simulink model "Refined_Model_40"  (R2020b)
settings: Solver=FixedStepAuto  StartTime=0.0  StopTime=5000  FixedStep=0.1  RelTol=1e-3
values from neighbouring files (symbols this model uses):
  ALInpSpeed = AxlLoss (1,:)    [GPS_val.m]    (also in ICEBEV_Script.m; ICEBEV_Script_VECTO.m; ICE_Script.m; ICE_Script_SSVal.m)
  ALInpTor = AxlLoss(:,1)    [GPS_val.m]    (also in ICEBEV_Script.m; ICEBEV_Script_VECTO.m; ICE_Script.m; ICE_Script_SSVal.m)
  ALTableVal = AxlLoss(2:end,2:end)    [GPS_val.m]    (also in ICEBEV_Script.m; ICEBEV_Script_VECTO.m; ICE_Script.m; ICE_Script_SSVal.m)
  CovDist = RoadProfile(:,4)    [ICE_Val.m]
  Cx = VehicleDefine(7,3)    [BEV_Basictest.m]    (also in GPS_val.m; ICEBEV_Script.m; ICEBEV_Script_VECTO.m; ICE_Script.m)
  Dist = 1:length(MaxSpeedProfile)    [GPS_val.m]    (also in ICE_Script.m; ICE_Val.m = [1:CovDist(end)])
  DynRolRad = VehicleDefine(5,3)    [BEV_Basictest.m]    (also in GPS_val.m; ICEBEV_Script.m; ICEBEV_Script_VECTO.m; ICE_Script.m)
  FDR = VehicleDefine(20,3)    [BEV_Basictest.m]    (also in GPS_val.m = VehicleDefine(22,3); ICEBEV_Script.m = VehicleDefine(22,3); ICEBEV_Script_VECTO.m = VehicleDefine(22,3); ICE_Script.m = VehicleDefine(22,3))
  Fr = VehicleDefine(13,3)    [BEV_Basictest.m]    (also in GPS_val.m; ICEBEV_Script.m; ICEBEV_Script_VECTO.m; ICE_Script.m)
  g = VehicleDefine(14,3)    [BEV_Basictest.m]    (also in GPS_val.m; ICEBEV_Script.m; ICEBEV_Script_VECTO.m; ICE_Script.m)
  GNo = GBXDefine(:,1)    [GPS_val.m]    (also in ICEBEV_Script.m; ICEBEV_Script_VECTO.m; ICE_Script.m; ICE_Script_SSVal.m)
  IntpSlope = round(IntpSlope,1)    [GPS_val.m]    (also in ICE_Script.m; ICE_Val.m = A)
  Jk = VehicleDefine(15,3)    [BEV_Basictest.m]    (also in GPS_val.m; ICEBEV_Script.m; ICEBEV_Script_VECTO.m; ICE_Script.m)
  MaxAcc = 1    [BEV_Basictest.m]    (also in GPS_val.m; ICEBEV_Script.m; ICEBEV_Script_VECTO.m; ICE_Script.m)
  MaxDec = 1    [BEV_Basictest.m]    (also in GPS_val.m; ICEBEV_Script.m; ICEBEV_Script_VECTO.m; ICE_Script.m)
  MaxSpeedProfile = FMSP    [GPS_val.m]    (also in ICE_Script.m; ICE_Val.m = repelem(SegSPLatinmps,SegLeninm))
  Me = VehicleDefine(10,3)    [BEV_Basictest.m]    (also in GPS_val.m; ICEBEV_Script.m; ICEBEV_Script_VECTO.m; ICE_Script.m)
  Mt = VehicleDefine(12,3)    [BEV_Basictest.m]    (also in GPS_val.m; ICEBEV_Script.m; ICEBEV_Script_VECTO.m; ICE_Script.m)
  Mtot = Mv+Me+Mt    [BEV_Basictest.m]    (also in GPS_val.m; ICEBEV_Script.m; ICEBEV_Script_VECTO.m; ICE_Script.m)
  Mv = VehicleDefine(9,3)    [BEV_Basictest.m]    (also in GPS_val.m; ICEBEV_Script.m; ICEBEV_Script_VECTO.m; ICE_Script.m)
  NoSteps = round(Dist(end))    [GPS_val.m]    (also in ICE_Script.m; ICE_Val.m = 3002)
  NoWhlFA = VehicleDefine(2,3)    [BEV_Basictest.m]    (also in GPS_val.m; ICE_Script.m; ICE_Val.m; ICE_Val_new.m)
  NoWhlRA = VehicleDefine(4,3)    [BEV_Basictest.m]    (also in GPS_val.m; ICE_Script.m; ICE_Val.m; ICE_Val_new.m)
  rho = VehicleDefine(6,3)    [BEV_Basictest.m]    (also in GPS_val.m; ICEBEV_Script.m; ICEBEV_Script_VECTO.m; ICE_Script.m)
  s = divisors(length(MaxSpeedProfile))    [GPS_val.m]    (also in ICEBEV_Script.m = round(FLoadTor); ICEBEV_Script_VECTO.m = round(FLoadTor); ICE_Script.m = round(FLoadTor); ICE_Script_SSVal.m = round(FLoadTor))
  SegNo = RoadProfile(:,1)    [ICE_Val.m]
  SegSPLatinmps = (sqrt(aMaxLat*g*CurRadinm))    [GPS_val.m]    (also in ICE_Script.m; ICE_Val.m)
  Sx = VehicleDefine(8,3)    [BEV_Basictest.m]    (also in GPS_val.m; ICEBEV_Script.m; ICEBEV_Script_VECTO.m; ICE_Script.m)
undefined symbols (not defined in the file or in its folder): G1Inprpm, Gmot, Jgbx, Stoptimes
libraries: autolibshared x2, vehdynlibtire x2, autolibdatasheetbattery x1, autolibmappedmotor x1
(part 3 of 3)

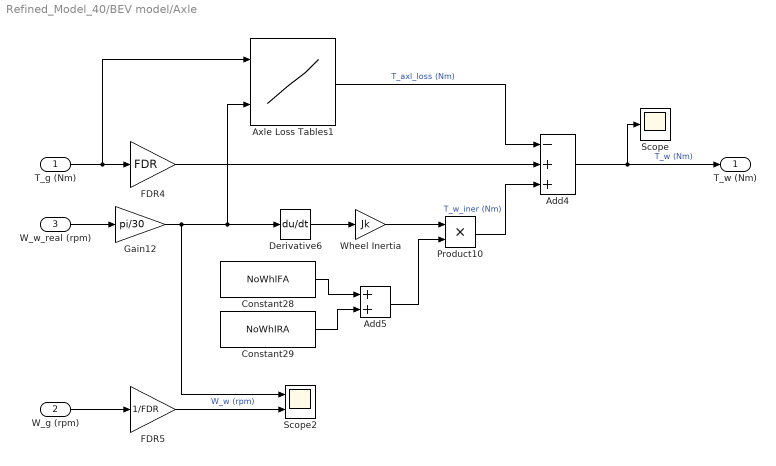
== system Refined_Model_40/BEV model/Axle ==
  T_g (Nm) : Inport
  W_g (rpm) : Inport  Port=2
  W_w_real (rpm) : Inport  Port=3
  Add4 : Sum  Inputs=-++
  Add5 : Sum
  Axle Loss Tables1 : Lookup_n-D  BreakpointsForDimension1=ALInpTor  BreakpointsForDimension2=ALInpSpeed  BreakpointsForDimension3=GNo  Table=ALTableVal  InterpMethod=Linear Lagrange  InternalRulePriority=Speed  RndMeth=Simplest  InputSameDT=on
      settings: InputPortMap=u0,u1
  Constant28 : Constant  Value=NoWhlFA
  Constant29 : Constant  Value=NoWhlRA
  Derivative6 : Derivative
  FDR4 : Gain  Gain=FDR
  FDR5 : Gain  Gain=1/FDR
  Gain12 : Gain  Gain=pi/30
  Product10 : Product
  Scope : Scope
  Scope2 : Scope  NumInputPorts=2
  Wheel Inertia : Gain  Gain=Jk
  T_w (Nm) : Outport
  wires:
  Product10/1 -> Add4/3  "T_w_iner (Nm)"
  Derivative6/1 -> Wheel Inertia/1
  Add5/1 -> Product10/2
  Constant29/1 -> Add5/2
  Constant28/1 -> Add5/1
  FDR4/1 -> Add4/2
  FDR5/1 -> Scope2/2  "W_w (rpm)"
  Wheel Inertia/1 -> Product10/1
  Add4/1 -> T_w (Nm)/1, Scope/1  "T_w (Nm)"
  T_g (Nm)/1 -> Axle Loss Tables1/1, FDR4/1
  W_g (rpm)/1 -> FDR5/1
  W_w_real (rpm)/1 -> Gain12/1
  Axle Loss Tables1/1 -> Add4/1  "T_axl_loss (Nm)"
  Gain12/1 -> Scope2/1, Axle Loss Tables1/2, Derivative6/1

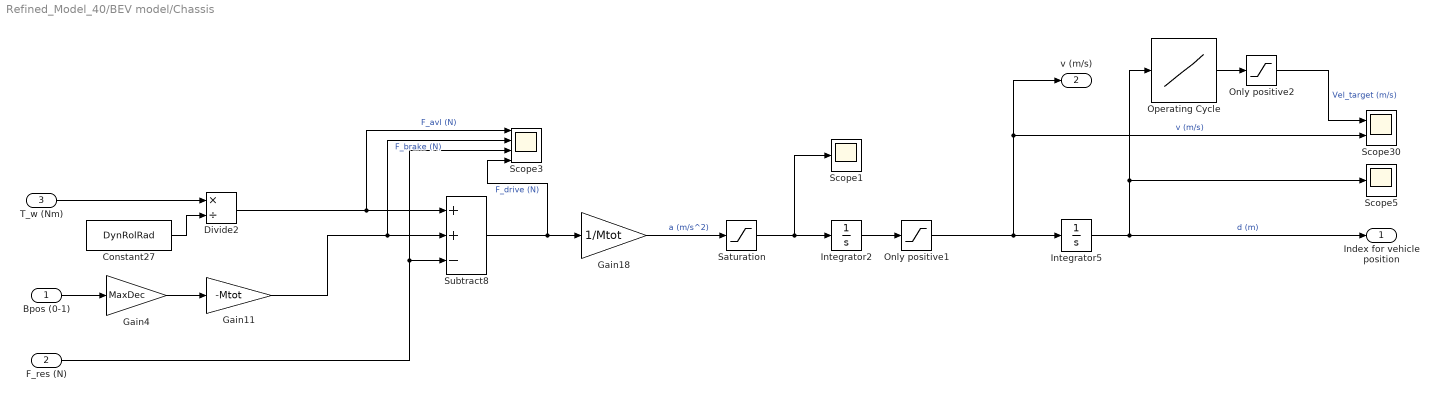
== system Refined_Model_40/BEV model/Chassis ==
  Bpos (0-1) : Inport
  F_res (N) : Inport  Port=2
  T_w (Nm) : Inport  Port=3
  Constant27 : Constant  Value=DynRolRad
  Divide2 : Product  Inputs=*/
  Gain11 : Gain  Gain=-Mtot
  Gain18 : Gain  Gain=1/Mtot
  Gain4 : Gain  Gain=MaxDec
  Integrator2 : Integrator  ContinuousStateAttributes='acceleration'
  Integrator5 : Integrator  ContinuousStateAttributes='velocity'
  Only positive1 : Saturate  UpperLimit=inf  LowerLimit=0
  Only positive2 : Saturate  UpperLimit=inf  LowerLimit=0
  Operating Cycle : Lookup_n-D  NumberOfTableDimensions=1  BreakpointsForDimension1=Dist  BreakpointsForDimension2=G1Inprpm  Table=MaxSpeedProfile  InterpMethod=Linear Lagrange  InternalRulePriority=Speed  RndMeth=Simplest  InputSameDT=on
  Saturation : Saturate  UpperLimit=MaxAcc  LowerLimit=-(MaxDec)
  Scope1 : Scope
  Scope3 : Scope  NumInputPorts=4
  Scope30 : Scope  NumInputPorts=2
  Scope5 : Scope
  Subtract8 : Sum  Inputs=++-
  Index for vehicle position : Outport
  v (m/s) : Outport  Port=2
  wires:
  Constant27/1 -> Divide2/2
  Subtract8/1 -> Scope3/4, Gain18/1  "F_drive (N)"
  Divide2/1 -> Subtract8/1, Scope3/1  "F_avl (N)"
  Integrator5/1 -> Index for vehicle position/1, Scope5/1, Operating Cycle/1  "d (m)"
  Integrator2/1 -> Only positive1/1
  T_w (Nm)/1 -> Divide2/1
  Gain11/1 -> Subtract8/2, Scope3/2  "F_brake (N)"
  Only positive1/1 -> v (m/s)/1, Scope30/2, Integrator5/1  "v (m/s)"
  Operating Cycle/1 -> Only positive2/1
  Gain18/1 -> Saturation/1  "a (m/s^2)"
  Bpos (0-1)/1 -> Gain4/1
  Gain4/1 -> Gain11/1
  F_res (N)/1 -> Subtract8/3, Scope3/3
  Saturation/1 -> Integrator2/1, Scope1/1
  Only positive2/1 -> Scope30/1  "Vel_target (m/s)"

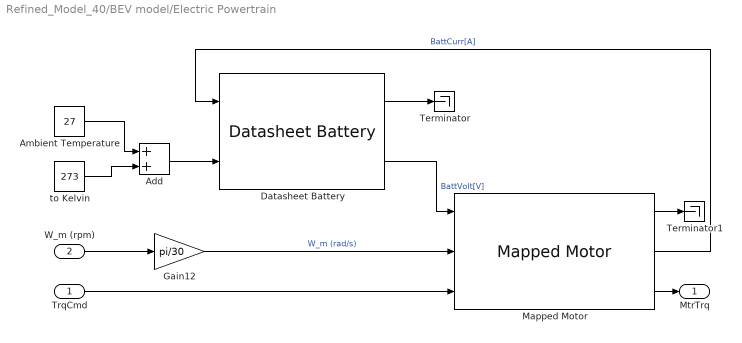
== system Refined_Model_40/BEV model/Electric Powertrain ==
  TrqCmd : Inport
  W_m (rpm) : Inport  Port=2
  Add : Sum
  Ambient Temperature : Constant  Value=27
  Datasheet Battery : autolibdatasheetbattery/Datasheet Battery  CapacityCtrl=Parameter  OutputVlt=Unfiltered  BattChargeMax=400  Em=[2.8 3.228 3.284 3.361 3.408 3.427 3.472 3.477 3.493 3.504 3.516 3.528 3.537 3.545 3.555 3.561 3.566 3.576 3.587 3.589 3.594 3.6 3.608 3.61 3.616 3.619 3.626 3.632 3.637 3.64 3.645 3.646 3.652 3.655 3.658 3.661 3.664 3.668 3.673 3.678 3.68 3.681 3.686 3.692 3.699 3.702 3.705 3.71 3.717 3.723 3.728 3.733 3.735 3.742 3.749 3.755 3.761 3.768 3.773 3.78 3.791 3.798 3.798 3.814 3.818 3.825 3.841 3.846 3.855 3.863 3.877 3.885 3.894 3.907 3.919 3.926 3.935 3.944 3.954 3.964 3.974 3.988 3.998 4.014 4.029 4.034 4.047 4.065 4.074 4.086 4.097 4.131 4.126 4.138 4.15 4.18 4.174 4.187 4.207 4.231 4.221]  CapLUTBp=[0 0.01 0.02 0.03 0.04 0.05 0.06 0.07 0.08 0.09 0.1 0.11 0.12 0.13 0.14 0.15 0.16 0.17 0.18 0.19 0.2 0.21 0.22 0.23 0.24 0.25 0.26 0.27 0.28 0.29 0.3 0.31 0.32 0.33 0.34 0.35 0.36 0.37 0.38 0.39 0.4 0.41 0.42 0.43 0.44 0.45 0.46 0.47 0.48 0.49 0.5 0.51 0.52 0.53 0.54 0.55 0.56 0.57 0.58 0.59 0.6 0.61 0.62 0.63 0.64 0.65 0.66 0.67 0.68 0.69 0.7 0.71 0.72 0.73 0.74 0.75 0.76 0.77 0.78 0.79 0.8 0.81 0.82 0.83 0.84 0.85 0.86 0.87 0.88 0.89 0.9 0.91 0.92 0.93 0.94 0.95 0.96 0.97 0.98 0.99 1]  RInt=[0.008846 0.009319 0.009027 0.00847 0.01032 0.01314;0.006389 0.006554 0.005553 0.005525 0.006043 0.007805;0.004364 0.004101 0.00406 0.003452 0.003846 0.004517;0.002031 0.002563 0.002532 0.00246 0.002716 0.003047;0.001443 0.001825 0.001795 0.001778 0.001924 0.002234;0.0005603 0.0007192 0.0006887 0.0007557 0.0007355 0.001014;0.001028 0.001338 0.001 0.001536 0.001546 0.002789]  BattTempBp=[243.1 253.1 263.1 273.1 283.1 298.1 313.1]  CapSOCBp=[0 0.2 0.4 0.6 0.8 1]  Ns=1  Np=1  BattCapInit=400  Tc=1/1000  Vinit=4.221  RefBlkName='autolibdatasheetbattery/Datasheet Battery'
      settings: SourceProductBaseCode=PW
  Gain12 : Gain  Gain=pi/30
  Mapped Motor : autolibmappedmotor/Mapped Motor  port_config=Speed  param_by=Maximum torque and power  w_t=[ 0 375 750 800 ]  T_t=[0.09 0.08 0.07 0]  torque_max=2200  power_max=295000  Tc=0.02  param_loss=Single efficiency measurement  eff=100  w_eff=375  T_eff=0.08  Piron=0  Pbase=0  w_eff_bp=[-8000 -4000 0 4000 8000]  T_eff_bp=[0 0.03 0.06 0.09]  Temp_eff_bp=[233.15 293.15 373.15]  losses_table=[1.49 1.67 2.21 3.10; 0.42 0.69 1.14 2.03; 0.06 0.24 0.78 1.68; 0.42 0.69 1.14 2.03; 1.49 1.67 2.21 3.10]  losses_table_3d=cat(3,1.05*[1.49 1.67 2.21 3.10; 0.42 0.69 1.14 2.03; 0.06 0.24 0.78 1.68; 0.42 0.69 1.14 2.03; 1.49 1.67 2.21 3.10],[1.49 1.67 2.21 3.10; 0.42 0.69 1.14 2.03; 0.06 0.24 0.78 1.68; 0.42 0.69 1.14 2.03; 1.49 1.67 2.21 3.10],1.03*[1.49 1.67 2.21 3.10; 0.42 0.69 1.14 2.03; 0.06 0.24 0.78 1.68; 0.42 0.69 1.14 2.03; 1.49 1.67 2.21 3.10])  efficiency_table=[95 95 95 95; 95 95 95 95; 95 95 95 95; 95 95 95 95; 95 95 95 95]  efficiency_table_3d=cat(3,90*ones(5,4),95*ones(5,4),92*ones(5,4))  J=5e-6  b=1e-5  omega_o=0  T_t_extended=[0 0.07 0.08 0.09 0.08 0.07 0]  w_t_extended=[-800 -750 -375 0 375 750 800]  KLossIron=0  KLossCopper=0  x_w_eff_vec=[-8000 -4000 0 4000 8000]  x_T_eff_vec=[-0.09 -0.06 -0.03 0 0.03 0.06 0.09]  x_tmp_eff_vec=[233.15 293.15 373.15]  x_losses_mat=[3.1 2.21 1.67 1.49 1.67 2.21 3.1;2.03 1.14 0.69 0.42 0.69 1.14 2.03;1.68 0.78 0.24 0.06 0.24 0.78 1.68;2.03 1.14 0.69 0.42 0.69 1.14 2.03;3.1 2.21 1.67 1.49 1.67 2.21 3.1]  x_losses_mat_3d=cat(3,[3.255 2.3205 1.7535 1.5645 1.7535 2.3205 3.255;2.1315 1.197 0.7245 0.441 0.7245 1.197 2.1315;1.764 0.819 0.252 0.063 0.252 0.819 1.764;2.1315 1.197 0.7245 0.441 0.7245 1.197 2.1315;3.255 2.3205 1.7535 1.5645 1.7535 2.3205 3.255],[3.1 2.21 1.67 1.49 1.67 2.21 3.1;2.03 1.14 0.69 0.42 0.69 1.14 2.03;1.68 0.78 0.24 0.06 0.24 0.78 1.68;2.03 1.14 0.69 0.42 0.69 1.14 2.03;3.1 2.21 1.67 1.49 1.67 2.21 3.1],[3.193 2.2763 1.7201 1.5347 1.7201 2.2763 3.193;2.0909 1.1742 0.7107 0.4326 0.7107 1.1742 2.0909;1.7304 0.8034 0.2472 0.0618 0.2472 0.8034 1.7304;2.0909 1.1742 0.7107 0.4326 0.7107 1.1742 2.0909;3.193 2.2763 1.7201 1.5347 1.7201 2.2763 3.193])  CalLossMapData={}  CalLossWithTempMapData={}  aMode=2  RefBlkName='autolibmappedmotor/Mapped Motor'
      settings: SourceProductBaseCode=PW,MT,UV,VE,VP
  Terminator : Terminator
  Terminator1 : Terminator
  to Kelvin : Constant  Value=273
  MtrTrq : Outport
  wires:
  Mapped Motor/3 -> MtrTrq/1
  Ambient Temperature/1 -> Add/1
  Datasheet Battery/2 -> Mapped Motor/1  "BattVolt[V]"
  W_m (rpm)/1 -> Gain12/1
  Mapped Motor/2 -> Datasheet Battery/1  "BattCurr[A]"
  to Kelvin/1 -> Add/2
  Add/1 -> Datasheet Battery/2
  TrqCmd/1 -> Mapped Motor/3
  Gain12/1 -> Mapped Motor/2  "W_m (rad/s)"
  Datasheet Battery/1 -> Terminator/1
  Mapped Motor/1 -> Terminator1/1

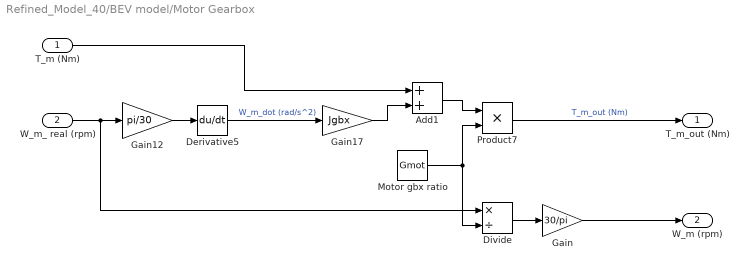
== system Refined_Model_40/BEV model/Motor Gearbox ==
  T_m (Nm) : Inport
  W_m_ real (rpm) : Inport  Port=2
  Add1 : Sum
  Derivative5 : Derivative
  Divide : Product  Inputs=*/
  Gain : Gain  Gain=30/pi
  Gain12 : Gain  Gain=pi/30
  Gain17 : Gain  Gain=Jgbx
  Motor gbx ratio : Constant  Value=Gmot
  Product7 : Product
  T_m_out (Nm) : Outport
  W_m (rpm) : Outport  Port=2
  wires:
  Motor gbx ratio/1 -> Product7/2, Divide/2
  Divide/1 -> Gain/1
  Gain/1 -> W_m (rpm)/1
  W_m_ real (rpm)/1 -> Divide/1, Gain12/1
  Add1/1 -> Product7/1
  Derivative5/1 -> Gain17/1  "W_m_dot (rad/s^2)"
  Gain17/1 -> Add1/2
  Product7/1 -> T_m_out (Nm)/1  "T_m_out (Nm)"
  T_m (Nm)/1 -> Add1/1
  Gain12/1 -> Derivative5/1

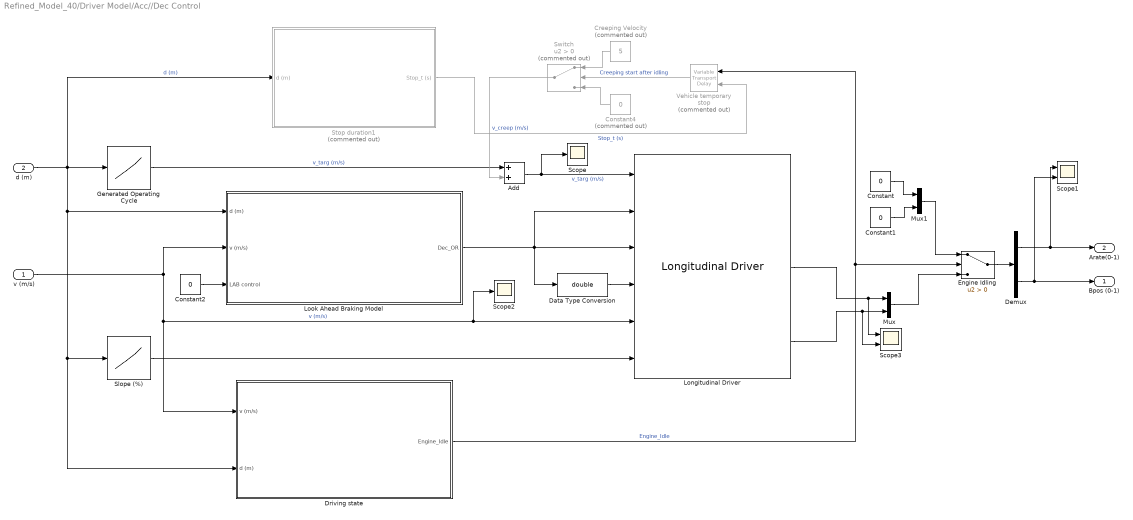
== system Refined_Model_40/Driver Model/Acc//Dec Control ==
  v (m/s) : Inport
  d (m) : Inport  Port=2
  Add : Sum
  Constant : Constant  Value=0
  Constant1 : Constant  Value=0
  Constant2 : Constant  Value=0
  Constant4 : Constant  Commented=on  Value=0
  Creeping Velocity : Constant  Commented=on  Value=5
  Data Type Conversion : DataTypeConversion  OutDataTypeStr=double
  Demux : Demux  Outputs=2
  Driving state : Subsystem
  Engine Idling : Switch  Criteria=u2 > Threshold
  Generated Operating Cycle : Lookup_n-D  NumberOfTableDimensions=1  BreakpointsForDimension1=Dist  BreakpointsForDimension2=G1Inprpm  Table=MaxSpeedProfile  InterpMethod=Linear Lagrange  InternalRulePriority=Speed  RndMeth=Simplest  InputSameDT=on
  Longitudinal Driver : autolibshared/Longitudinal Driver  extAccelOvr=off  extDecelOvr=on  extAccelHld=off  extDecelHld=off  extAccelZero=on  extDecelZero=off  cntrlType=PI  shftType=None  velUnits=m/s  gearOut=off  Kp=1  Ki=1  Kff=0  Kg=0  VehVelVec=[0 100]  KffVec=[.1 .1]  KpVec=[10 10]  KiVec=[5 5]  KgVec=[0 0]  m=1500  Kpt=3000  tau=.1  L=2  aR=200  bR=2.5  cR=.5  g=9.81  vnom=100  Kaw=0  tauerr=0  tauPt=2  GearInit=0  tShift=.1  pdlVec=[0.1 0.4 0.5 0.9]  upShftTbl=[-1 12.9375 26.4375 39.9375 51.18749999999999 62.4375 72.84375 83.25;-1 16.3125 29.8125 43.3125 54.5624 65.8125 76.78125 87.75;-1 19.6875 33.1875 46.68749999999999 57.9375 69.1875 80.71875 92.25;-1 33 52.5 77.25 100.5 138.75 161.875 185]  dwnShftTbl=[1 9.5625 23.0625 36.5625 47.8125 59.0625 68.90625 78.75;1 12.9375 26.4375 39.9375 51.18749999999999 62.4375 72.84375 83.25;1 16.3125 29.8125 43.3125 54.562499 65.8125 76.78125 87.75;1 19.6875 33.1875 46.68749999999999 57.9375 69.1875 80.71875 92.25]  tClutch=.5  tRev=.5  tPark=120  aMode=1  UpGearVec="[0  1  2  3  4  5  6  7]"  DownGearVec="[1  2  3  4  5  6  7  8]"
      settings: SourceProductBaseCode=PW,MT,UV,VE,VP
  Look Ahead Braking Model : Subsystem
  Mux : Mux  Inputs=2
  Mux1 : Mux  Inputs=2
  Scope : Scope
  Scope1 : Scope  NumInputPorts=2
  Scope2 : Scope
  Scope3 : Scope  NumInputPorts=2
  Slope (%) : Lookup_n-D  NumberOfTableDimensions=1  BreakpointsForDimension1=Dist  Table=IntpSlope  InternalRulePriority=Speed  RndMeth=Simplest  InputSameDT=on
  Stop duration1 : Subsystem  Commented=on
  Switch : Switch  Commented=on  Criteria=u2 > Threshold
  Vehicle temporary stop : VariableTransportDelay  Commented=on  VariableDelayType=Variable transport delay  MaximumDelay=10
  Bpos (0-1) : Outport
  Arate(0-1) : Outport  Port=2
  wires:
  Add/1 -> Scope/1, Longitudinal Driver/1  "v_targ (m/s)"
  Slope (%)/1 -> Longitudinal Driver/6
  Demux/1 -> Scope1/1, Arate(0-1)/1
  Demux/2 -> Bpos (0-1)/1, Scope1/2
  Constant/1 -> Mux1/1
  Mux/1 -> Engine Idling/3
  Constant1/1 -> Mux1/2
  Mux1/1 -> Engine Idling/1
  Engine Idling/1 -> Demux/1
  d (m)/1 -> Stop duration1/1(d (m)), Driving state/2(d (m)), Slope (%)/1, Look Ahead Braking Model/1(d (m)), Generated Operating Cycle/1  "d (m)"
  v (m/s)/1 -> Scope2/1, Longitudinal Driver/5, Driving state/1(v (m/s)), Look Ahead Braking Model/2(v (m/s))  "v (m/s)"
  Generated Operating Cycle/1 -> Add/1  "v_targ (m/s)"
  Data Type Conversion/1 -> Longitudinal Driver/4
  Longitudinal Driver/3 -> Scope3/2, Mux/2
  Stop duration1/1(Stop_t (s)) -> Vehicle temporary stop/2  "Stop_t (s)"
  Driving state/1(Engine_Idle) -> Vehicle temporary stop/1, Engine Idling/2  "Engine_Idle"
  Creeping Velocity/1 -> Switch/1
  Constant4/1 -> Switch/3
  Vehicle temporary stop/1 -> Switch/2  "Creeping start after idling"
  Switch/1 -> Add/2  "v_creep (m/s)"
  Look Ahead Braking Model/1(Dec_OR) -> Longitudinal Driver/2, Longitudinal Driver/3, Data Type Conversion/1
  Longitudinal Driver/2 -> Mux/1, Scope3/1
  Constant2/1 -> Look Ahead Braking Model/3(LAB control)

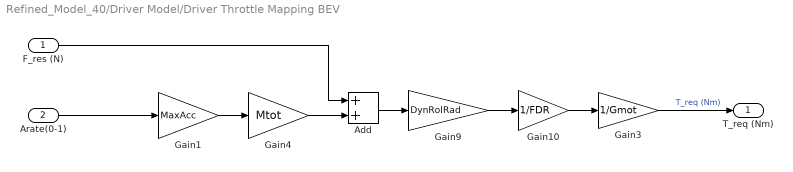
== system Refined_Model_40/Driver Model/Driver Throttle Mapping BEV ==
  F_res (N) : Inport
  Arate(0-1) : Inport  Port=2
  Add : Sum
  Gain1 : Gain  Gain=MaxAcc
  Gain10 : Gain  Gain=1/FDR
  Gain3 : Gain  Gain=1/Gmot
  Gain4 : Gain  Gain=Mtot
  Gain9 : Gain  Gain=DynRolRad
  T_req (Nm) : Outport
  wires:
  Gain3/1 -> T_req (Nm)/1  "T_req (Nm)"
  Gain1/1 -> Gain4/1
  Gain9/1 -> Gain10/1
  Add/1 -> Gain9/1
  Gain4/1 -> Add/2
  Gain10/1 -> Gain3/1
  F_res (N)/1 -> Add/1
  Arate(0-1)/1 -> Gain1/1

== system Refined_Model_40/Environment/If Action Subsystem ==
  In1 : Inport
  Action Port : ActionPort  ActionPortLabel=if(u1 > 0)
  Out1 : Outport
  wires:
  In1/1 -> Out1/1

== system Refined_Model_40/Environment/If Action Subsystem1 ==
  In1 : Inport
  Action Port : ActionPort  ActionPortLabel=else
  Out1 : Outport
  wires:
  In1/1 -> Out1/1

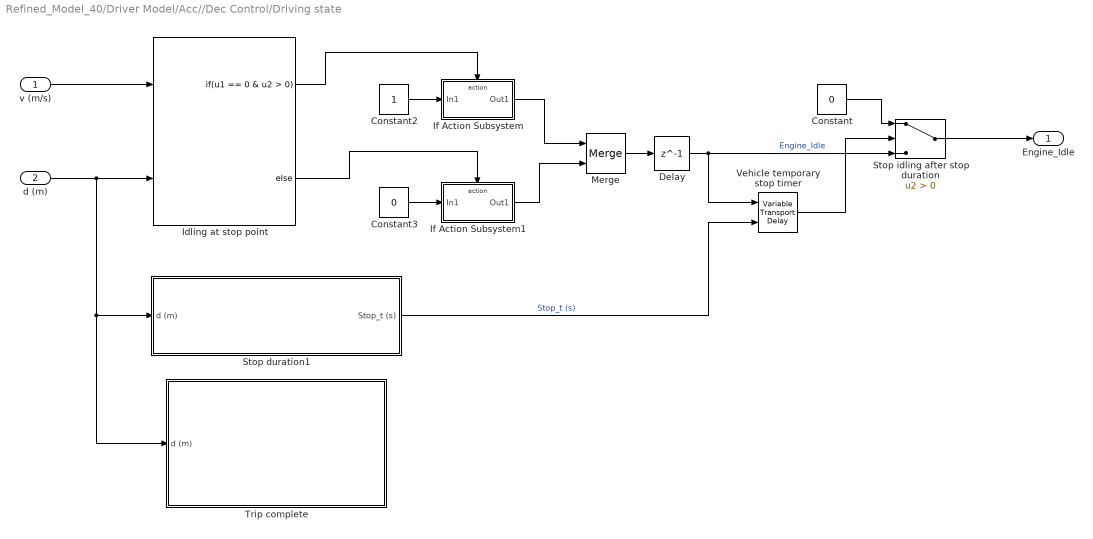
== system Refined_Model_40/Driver Model/Acc//Dec Control/Driving state ==
  v (m/s) : Inport
  d (m) : Inport  Port=2
  Constant : Constant  Value=0
  Constant2 : Constant
  Constant3 : Constant  Value=0
  Delay : Delay  DelayLength=1
  Idling at stop point : If  NumInputs=2  IfExpression=u1 == 0 & u2 > 0
  If Action Subsystem : Subsystem  TreatAsAtomicUnit=on
  If Action Subsystem1 : Subsystem  TreatAsAtomicUnit=on
  Merge : Merge
  Stop duration1 : Subsystem
  Stop idling after stop duration : Switch  Criteria=u2 > Threshold
  Trip complete : Subsystem
  Vehicle temporary stop timer : VariableTransportDelay  VariableDelayType=Variable transport delay  MaximumDelay=10
  Engine_Idle : Outport
  wires:
  Constant2/1 -> If Action Subsystem/1(In1)
  If Action Subsystem/1(Out1) -> Merge/1
  Merge/1 -> Delay/1
  Idling at stop point/1 -> If Action Subsystem/Action
  Constant3/1 -> If Action Subsystem1/1(In1)
  Idling at stop point/2 -> If Action Subsystem1/Action
  If Action Subsystem1/1(Out1) -> Merge/2
  v (m/s)/1 -> Idling at stop point/1
  d (m)/1 -> Trip complete/1(d (m)), Stop duration1/1(d (m)), Idling at stop point/2
  Constant/1 -> Stop idling after stop duration/1
  Stop duration1/1(Stop_t (s)) -> Vehicle temporary stop timer/2  "Stop_t (s)"
  Vehicle temporary stop timer/1 -> Stop idling after stop duration/2
  Delay/1 -> Vehicle temporary stop timer/1, Stop idling after stop duration/3  "Engine_Idle"
  Stop idling after stop duration/1 -> Engine_Idle/1

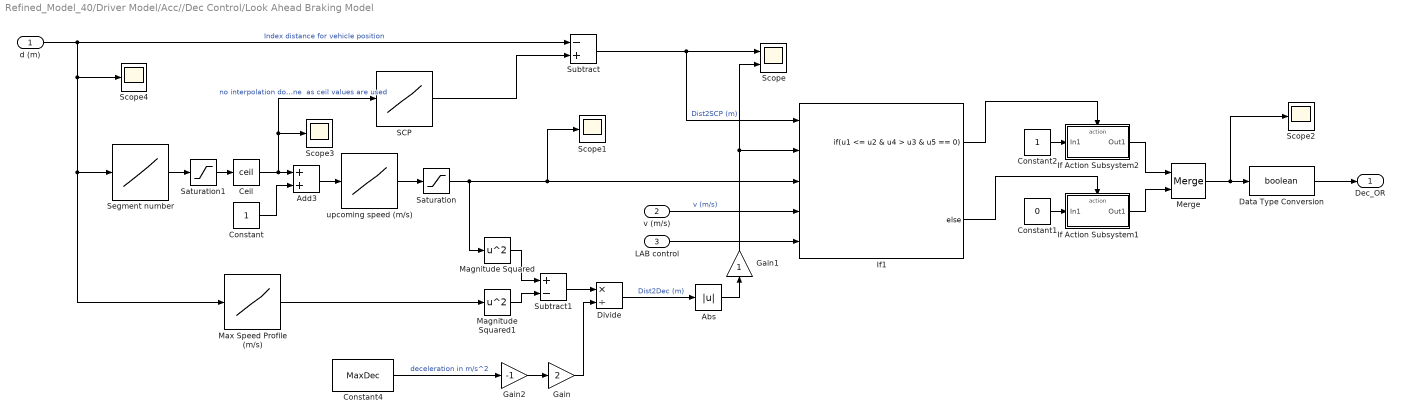
== system Refined_Model_40/Driver Model/Acc//Dec Control/Look Ahead Braking Model ==
  d (m) : Inport
  v (m/s) : Inport  Port=2
  LAB control : Inport  Port=3
  Abs : Abs
  Add3 : Sum
  Ceil : Rounding  Operator=ceil
  Constant : Constant
  Constant1 : Constant  Value=0
  Constant2 : Constant
  Constant4 : Constant  Value=MaxDec
  Data Type Conversion : DataTypeConversion  OutDataTypeStr=boolean
  Divide : Product  Inputs=*/
  Gain : Gain  Gain=2
  Gain1 : Gain
  Gain2 : Gain  Gain=-1
  If Action Subsystem1 : Subsystem  TreatAsAtomicUnit=on
  If Action Subsystem2 : Subsystem  TreatAsAtomicUnit=on
  If1 : If  NumInputs=5  IfExpression=u1 <= u2 & u4 > u3 & u5 == 0
  Magnitude Squared : Math  Operator=square  SaturateOnIntegerOverflow=on
  Magnitude Squared1 : Math  Operator=square  SaturateOnIntegerOverflow=on
  Max Speed Profile (m/s) : Lookup_n-D  NumberOfTableDimensions=1  BreakpointsForDimension1=Dist  BreakpointsForDimension2=G1Inprpm  Table=MaxSpeedProfile  InterpMethod=Linear Lagrange  InternalRulePriority=Speed  RndMeth=Simplest  InputSameDT=on
  Merge : Merge
  SCP : Lookup_n-D  NumberOfTableDimensions=1  BreakpointsForDimension1=SegNo  BreakpointsForDimension2=G1Inprpm  Table=CovDist  InterpMethod=Linear Lagrange  InternalRulePriority=Speed  RndMeth=Simplest  InputSameDT=on
  Saturation : Saturate  UpperLimit=inf  LowerLimit=0
  Saturation1 : Saturate  UpperLimit=inf  LowerLimit=0
  Scope : Scope  NumInputPorts=2
  Scope{1..4} (4 alike) : Scope
  Segment number : Lookup_n-D  NumberOfTableDimensions=1  BreakpointsForDimension1=CovDist  BreakpointsForDimension2=G1Inprpm  Table=SegNo  InterpMethod=Linear Lagrange  InternalRulePriority=Speed  RndMeth=Simplest  InputSameDT=on
  Subtract : Sum  Inputs=-+
  Subtract1 : Sum  Inputs=+-
  upcoming speed (m/s) : Lookup_n-D  NumberOfTableDimensions=1  BreakpointsForDimension1=SegNo  BreakpointsForDimension2=G1Inprpm  Table=SegSPLatinmps  InterpMethod=Linear Lagrange  InternalRulePriority=Speed  RndMeth=Simplest  InputSameDT=on
  Dec_OR : Outport
  wires:
  Add3/1 -> upcoming speed (m/s)/1
  Ceil/1 -> Add3/1, Scope3/1, SCP/1  "no interpolation done  as ceil values are used"
  SCP/1 -> Subtract/2
  Constant/1 -> Add3/2
  Subtract/1 -> Scope/1, If1/1  "Dist2SCP (m)"
  Segment number/1 -> Saturation1/1
  Magnitude Squared/1 -> Subtract1/1
  Constant4/1 -> Gain2/1  "deceleration in m/s^2"
  Divide/1 -> Abs/1  "Dist2Dec (m)"
  Constant1/1 -> If Action Subsystem1/1(In1)
  Constant2/1 -> If Action Subsystem2/1(In1)
  If1/1 -> If Action Subsystem2/Action
  If Action Subsystem2/1(Out1) -> Merge/1
  Magnitude Squared1/1 -> Subtract1/2
  Merge/1 -> Scope2/1, Data Type Conversion/1
  Data Type Conversion/1 -> Dec_OR/1
  Max Speed Profile (m/s)/1 -> Magnitude Squared1/1
  d (m)/1 -> Subtract/1, Scope4/1, Segment number/1, Max Speed Profile (m/s)/1  "Index distance for vehicle position"
  Subtract1/1 -> Divide/1
  Gain2/1 -> Gain/1
  Gain/1 -> Divide/2
  If1/2 -> If Action Subsystem1/Action
  If Action Subsystem1/1(Out1) -> Merge/2
  Abs/1 -> Gain1/1
  Gain1/1 -> Scope/2, If1/2
  v (m/s)/1 -> If1/4  "v (m/s)"
  upcoming speed (m/s)/1 -> Saturation/1
  Saturation/1 -> Scope1/1, If1/3, Magnitude Squared/1
  LAB control/1 -> If1/5
  Saturation1/1 -> Ceil/1

== system Refined_Model_40/Driver Model/Acc//Dec Control/Stop duration1 ==
  d (m) : Inport
  1-D Lookup Table : Lookup_n-D  NumberOfTableDimensions=1  BreakpointsForDimension1=Stoptimes(:,1)  Table=1:length(Stoptimes)  InternalRulePriority=Speed  RndMeth=Simplest  InputSameDT=on
  Ceil : Rounding  Operator=ceil
  Constant2 : Constant
  Direct Lookup Table (n-D) : LookupNDDirect  NumberOfTableDimensions=1  Table=Stoptimes(:,2)
  Scope : Scope
  Subtract1 : Sum  Inputs=+-
  Stop_t (s) : Outport
  wires:
  1-D Lookup Table/1 -> Ceil/1
  d (m)/1 -> 1-D Lookup Table/1
  Subtract1/1 -> Direct Lookup Table (n-D)/1
  Direct Lookup Table (n-D)/1 -> Stop_t (s)/1, Scope/1  "Stop time (s)"
  Ceil/1 -> Subtract1/1
  Constant2/1 -> Subtract1/2

== system Refined_Model_40/Driver Model/Acc//Dec Control/Driving state/If Action Subsystem ==
  In1 : Inport
  Action Port : ActionPort  ActionPortLabel=if(u1 == 0 & u2 > 0)
  Out1 : Outport
  wires:
  In1/1 -> Out1/1

== system Refined_Model_40/Driver Model/Acc//Dec Control/Driving state/If Action Subsystem1 ==
  In1 : Inport
  Action Port : ActionPort  ActionPortLabel=else
  Out1 : Outport
  wires:
  In1/1 -> Out1/1

== system Refined_Model_40/Driver Model/Acc//Dec Control/Driving state/Stop duration1 ==
  d (m) : Inport
  1-D Lookup Table : Lookup_n-D  NumberOfTableDimensions=1  BreakpointsForDimension1=Stoptimes(:,1)  Table=1:length(Stoptimes)  InternalRulePriority=Speed  RndMeth=Simplest  InputSameDT=on
  Ceil : Rounding  Operator=ceil
  Constant2 : Constant
  Direct Lookup Table (n-D) : LookupNDDirect  NumberOfTableDimensions=1  Table=Stoptimes(:,2)
  Scope : Scope
  Subtract1 : Sum  Inputs=+-
  Stop_t (s) : Outport
  wires:
  1-D Lookup Table/1 -> Ceil/1
  d (m)/1 -> 1-D Lookup Table/1
  Subtract1/1 -> Direct Lookup Table (n-D)/1
  Direct Lookup Table (n-D)/1 -> Stop_t (s)/1, Scope/1  "Stop time (s)"
  Ceil/1 -> Subtract1/1
  Constant2/1 -> Subtract1/2

== system Refined_Model_40/Driver Model/Acc//Dec Control/Driving state/Trip complete ==
  d (m) : Inport
  Constant1 : Constant  Value=NoSteps
  Constant2 : Constant
  Delay : Delay  DelayLength=1
  Derivative : Derivative
  If : If  NumInputs=3  IfExpression=u1 > u2 & u3 ==0  ShowElse=off
  If Action Subsystem : Subsystem  TreatAsAtomicUnit=on
  Stop Simulation : Stop
  wires:
  Constant1/1 -> If/2
  Constant2/1 -> If Action Subsystem/1(In1)
  If/1 -> If Action Subsystem/Action
  If Action Subsystem/1(Out1) -> Delay/1
  d (m)/1 -> If/1, Derivative/1
  Delay/1 -> Stop Simulation/1
  Derivative/1 -> If/3  "v (m/s)"

== system Refined_Model_40/Driver Model/Acc//Dec Control/Look Ahead Braking Model/If Action Subsystem1 ==
  In1 : Inport
  Action Port : ActionPort  ActionPortLabel=else
  Out1 : Outport
  wires:
  In1/1 -> Out1/1

== system Refined_Model_40/Driver Model/Acc//Dec Control/Look Ahead Braking Model/If Action Subsystem2 ==
  In1 : Inport
  Action Port : ActionPort  ActionPortLabel=if(u1 <= u2 & u4 > u3 & u5 == 0)
  Out1 : Outport
  wires:
  In1/1 -> Out1/1

== system Refined_Model_40/Driver Model/Acc//Dec Control/Driving state/Trip complete/If Action Subsystem ==
  In1 : Inport
  Action Port : ActionPort  ActionPortLabel=if(u1 > u2 & u3 ==0)
  Out1 : Outport
  wires:
  In1/1 -> Out1/1
